simulink model "purple_noise"  (R2023b)
settings: Solver=VariableStepAuto  StartTime=0.0  StopTime=10.0  RelTol=1e-3
settings Model: Creator=awcm9  LastModifiedBy=awcm9

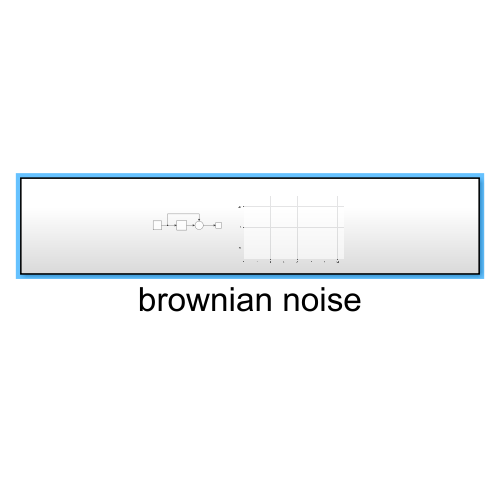
[thumbnail: Simulink's stored preview of the top-level diagram]
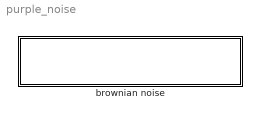
== system purple_noise ==
  brownian noise : Subsystem

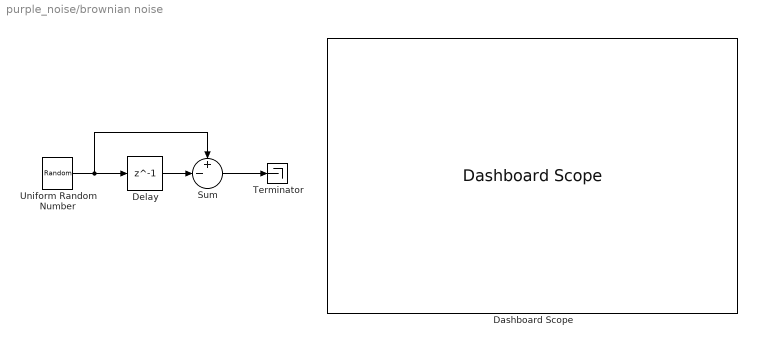
== system purple_noise/brownian noise ==
  Dashboard Scope : DashboardScope  ShowInitialText=off  TimeSpan=15  Ymin=-30  Ymax=30  ScaleAtStop=off
  Delay : Delay  DelayLength=1
  Sum : Sum  Inputs=+-|
  Terminator : Terminator
  Uniform Random Number : UniformRandomNumber  SampleTime=1
  wires:
  Sum/1 -> Terminator/1
  Delay/1 -> Sum/2
  Uniform Random Number/1 -> Delay/1, Sum/1
